simulink model "main"  (R2024a)
settings: Solver=VariableStepAuto  StartTime=0.0  StopTime=stop_time  RelTol=1e-3
values from neighbouring files (symbols this model uses):
  A_ca = sqrt(2)    [load_params.m]
  c = 299792458    [load_params.m]
  ca_code = 1    [load_params.m]
  code_repeat = 0.001    [load_params.m]
  data_repeat = 30    [load_params.m]
  df_Dop = 0    [load_params.m]
  dt_iono = 0    [load_params.m]
  dt_rec = 0.001    [load_params.m]
  dt_sv = 0    [load_params.m]
  dt_tropo = 0    [load_params.m]
  fB = 1.5e6    (= 1500000)    [load_params.m]
  fb = fB    (= 1500000)    [load_params.m]
  fc = 1.023e6    (= 1023000)    [load_params.m]
  fdata = 50    [load_params.m]
  ferr = 0    [load_params.m]
  fL1 = 1575.42e6    (= 1575420000)    [load_params.m]
  fs = 4e6    (= 4000000)    [load_params.m]
  nav_data = 1    [load_params.m]
  perr_rad = 0    [load_params.m]
  PIT = 0.010    (= 0.01)    [load_params.m]
  r_true_t0 = 20e6    (= 20000000)    [load_params.m]
  Ts = 1/fs    (= 2.5e-07)    [load_params.m]
undefined symbols (not defined in the file or in its folder): DiscIntNeverNeededParam
libraries: dspsrcs4 x2, commfilt2 x2
settings Model: Creator=Alireza  LastModifiedBy=Alireza

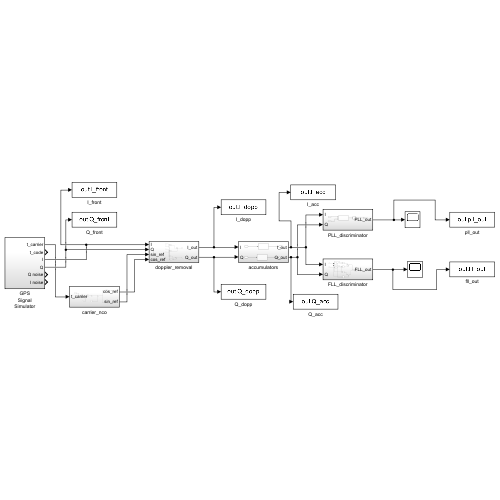
[thumbnail: Simulink's stored preview of the top-level diagram]
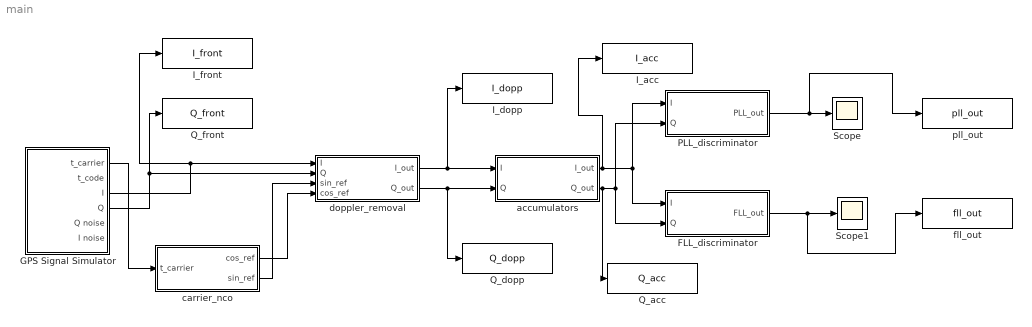
== system main ==
  FLL_discriminator : Subsystem
  GPS Signal Simulator : Subsystem
  I_acc : ToWorkspace  VariableName=I_acc  SampleTime=-1
  I_dopp : ToWorkspace  VariableName=I_dopp  SampleTime=-1
  I_front : ToWorkspace  VariableName=I_front  SampleTime=-1
  PLL_discriminator : Subsystem
  Q_acc : ToWorkspace  VariableName=Q_acc  SampleTime=-1
  Q_dopp : ToWorkspace  VariableName=Q_dopp  SampleTime=-1
  Q_front : ToWorkspace  VariableName=Q_front  SampleTime=-1
  Scope : Scope
  Scope1 : Scope
  accumulators : Subsystem
  carrier_nco : Subsystem
  doppler_removal : Subsystem
  fll_out : ToWorkspace  VariableName=fll_out  SampleTime=-1
  pll_out : ToWorkspace  VariableName=pll_out  SampleTime=-1
  wires:
  carrier_nco/1(cos_ref) -> doppler_removal/4(cos_ref)
  carrier_nco/2(sin_ref) -> doppler_removal/3(sin_ref)
  doppler_removal/1(I_out) -> I_dopp/1, accumulators/1(I)
  doppler_removal/2(Q_out) -> Q_dopp/1, accumulators/2(Q)
  accumulators/1(I_out) -> I_acc/1, FLL_discriminator/1(I), PLL_discriminator/1(I)
  accumulators/2(Q_out) -> Q_acc/1, FLL_discriminator/2(Q), PLL_discriminator/2(Q)
  GPS Signal Simulator/3(I) -> I_front/1, doppler_removal/1(I)
  GPS Signal Simulator/4(Q) -> Q_front/1, doppler_removal/2(Q)
  GPS Signal Simulator/1(t_carrier) -> carrier_nco/1(t_carrier)
  PLL_discriminator/1(PLL_out) -> pll_out/1, Scope/1
  FLL_discriminator/1(FLL_out) -> fll_out/1, Scope1/1

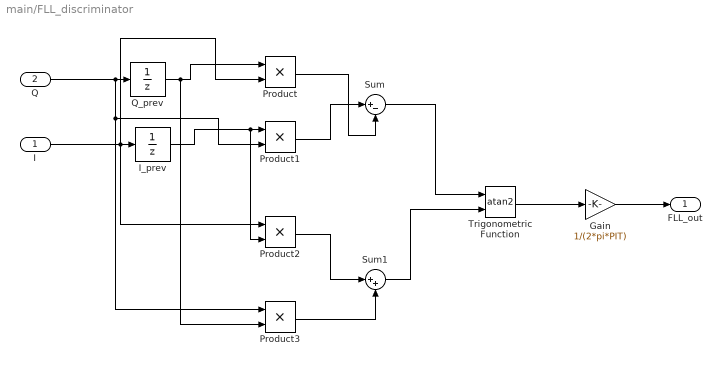
== system main/FLL_discriminator ==
  I : Inport
  Q : Inport  Port=2
  Gain : Gain  Gain=1/(2*pi*PIT)
  I_prev : UnitDelay  SampleTime=-1  HasFrameUpgradeWarning=on
  Product{,1..3} (4 alike) : Product
  Q_prev : UnitDelay  SampleTime=-1  HasFrameUpgradeWarning=on
  Sum : Sum  Inputs=|+-
  Sum1 : Sum  Inputs=|++
  Trigonometric Function : Trigonometry  Operator=atan2
  FLL_out : Outport
  wires:
  I/1 -> Product/2, I_prev/1, Product2/1
  Q/1 -> Product1/2, Product3/1, Q_prev/1
  I_prev/1 -> Product2/2, Product1/1
  Q_prev/1 -> Product3/2, Product/1
  Product1/1 -> Sum/1
  Product/1 -> Sum/2
  Product2/1 -> Sum1/1
  Product3/1 -> Sum1/2
  Sum/1 -> Trigonometric Function/1
  Sum1/1 -> Trigonometric Function/2
  Trigonometric Function/1 -> Gain/1
  Gain/1 -> FLL_out/1

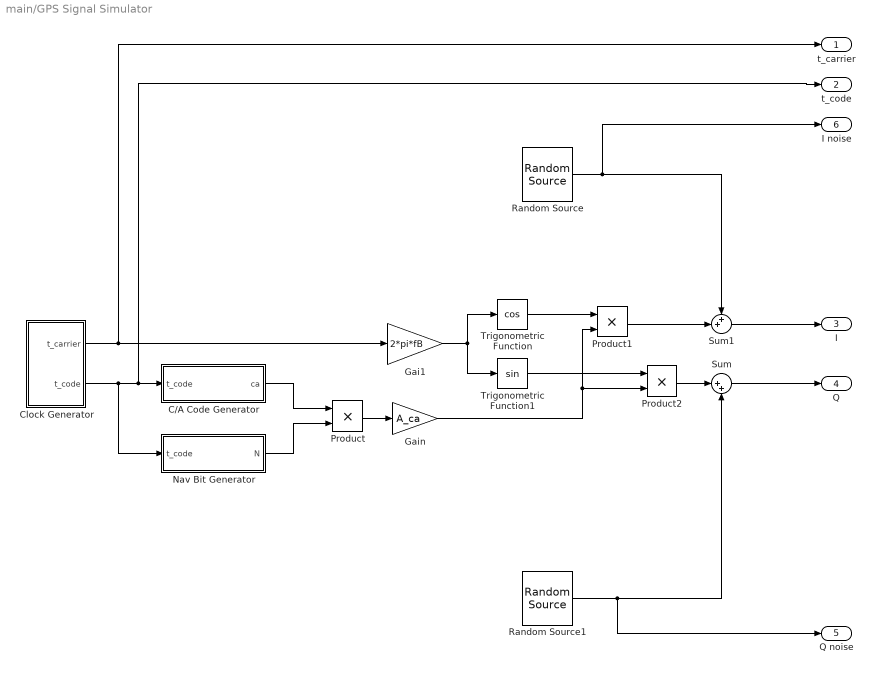
== system main/GPS Signal Simulator ==
  C/A Code Generator : Subsystem
  Clock Generator : Subsystem
  Gai1 : Gain  Gain=2*pi*fB
  Gain : Gain  Gain=A_ca
  Nav Bit Generator : Subsystem
  Product : Product  RndMeth=Zero
  Product1 : Product  RndMeth=Zero
  Product2 : Product  RndMeth=Zero
  Random Source : dspsrcs4/Random Source  SrcType=Gaussian  MinVal=0  MaxVal=1  MeanVal=0  VarVal=Pn  RepMode=Specify seed  rawSeed=1  IsInherit=off  SampTime=Ts  SampFrame=1  OutComplex=Real  DataType=double  SimulateUsing=Interpreted execution
  Random Source1 : dspsrcs4/Random Source  SrcType=Gaussian  MinVal=0  MaxVal=1  MeanVal=0  VarVal=Pn  RepMode=Specify seed  rawSeed=2  IsInherit=off  SampTime=Ts  SampFrame=1  OutComplex=Real  DataType=double  SimulateUsing=Interpreted execution
  Sum : Sum  Inputs=|++
  Sum1 : Sum  Inputs=++|
  Trigonometric Function : Trigonometry  Operator=cos
  Trigonometric Function1 : Trigonometry
  t_carrier : Outport
  t_code : Outport  Port=2
  I : Outport  Port=3
  Q : Outport  Port=4
  Q noise : Outport  Port=5
  I noise : Outport  Port=6
  wires:
  Clock Generator/2(t_code) -> Nav Bit Generator/1(t_code), C/A Code Generator/1(t_code), t_code/1
  C/A Code Generator/1(ca) -> Product/1
  Nav Bit Generator/1(N) -> Product/2
  Product/1 -> Gain/1
  Clock Generator/1(t_carrier) -> Gai1/1, t_carrier/1
  Gai1/1 -> Trigonometric Function1/1, Trigonometric Function/1
  Gain/1 -> Product1/2, Product2/2
  Trigonometric Function/1 -> Product1/1
  Trigonometric Function1/1 -> Product2/1
  Random Source1/1 -> Sum/2, Q noise/1
  Random Source/1 -> Sum1/1, I noise/1
  Sum/1 -> Q/1
  Sum1/1 -> I/1
  Product1/1 -> Sum1/2
  Product2/1 -> Sum/1

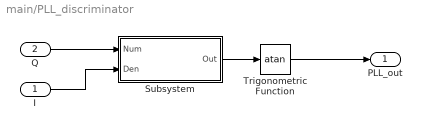
== system main/PLL_discriminator ==
  I : Inport
  Q : Inport  Port=2
  Subsystem : Subsystem
  Trigonometric Function : Trigonometry  Operator=atan
  PLL_out : Outport
  wires:
  Subsystem/1(Out) -> Trigonometric Function/1
  Trigonometric Function/1 -> PLL_out/1
  Q/1 -> Subsystem/1(Num)
  I/1 -> Subsystem/2(Den)

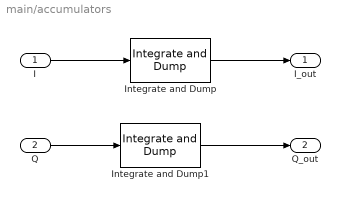
== system main/accumulators ==
  I : Inport
  Q : Inport  Port=2
  Integrate and Dump : commfilt2/Integrate and Dump  obssamples=PIT*fs  offsetsamples=0  nodump=off  roundingMode=Floor  overflowMode=off  outputDataTypeStr=Inherit: Same as accumulator  outputLastDataTypeStr=Inherit: Same as accumulator
  Integrate and Dump1 : commfilt2/Integrate and Dump  obssamples=PIT*fs  offsetsamples=0  nodump=off  roundingMode=Floor  overflowMode=off  outputDataTypeStr=Inherit: Same as accumulator  outputLastDataTypeStr=Inherit: Same as accumulator
  I_out : Outport
  Q_out : Outport  Port=2
  wires:
  I/1 -> Integrate and Dump/1
  Integrate and Dump/1 -> I_out/1
  Integrate and Dump1/1 -> Q_out/1
  Q/1 -> Integrate and Dump1/1

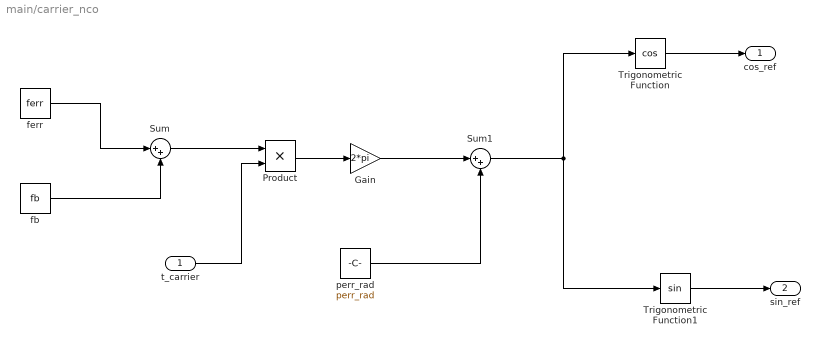
== system main/carrier_nco ==
  t_carrier : Inport
  Gain : Gain  Gain=2*pi
  Product : Product
  Sum : Sum  Inputs=|++
  Sum1 : Sum  Inputs=|++
  Trigonometric Function : Trigonometry  Operator=cos
  Trigonometric Function1 : Trigonometry
  fb : Constant  Value=fb
  ferr : Constant  Value=ferr
  perr_rad : Constant  Value=perr_rad
  cos_ref : Outport
  sin_ref : Outport  Port=2
  wires:
  Trigonometric Function1/1 -> sin_ref/1
  t_carrier/1 -> Product/2
  Sum1/1 -> Trigonometric Function1/1, Trigonometric Function/1
  Trigonometric Function/1 -> cos_ref/1
  perr_rad/1 -> Sum1/2
  Gain/1 -> Sum1/1
  fb/1 -> Sum/2
  Product/1 -> Gain/1
  ferr/1 -> Sum/1
  Sum/1 -> Product/1

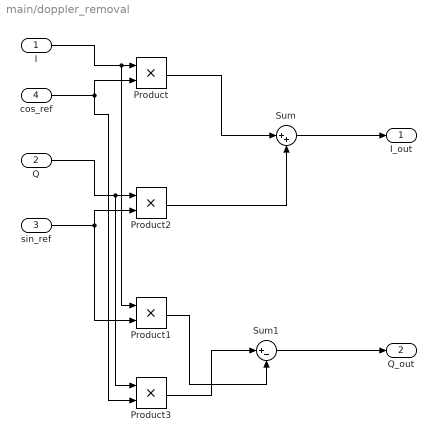
== system main/doppler_removal ==
  I : Inport
  Q : Inport  Port=2
  sin_ref : Inport  Port=3
  cos_ref : Inport  Port=4
  Product{,1..3} (4 alike) : Product
  Sum : Sum  Inputs=|++
  Sum1 : Sum  Inputs=|+-
  I_out : Outport
  Q_out : Outport  Port=2
  wires:
  I/1 -> Product1/1, Product/1
  cos_ref/1 -> Product3/2, Product/2
  Q/1 -> Product2/1, Product3/1
  sin_ref/1 -> Product1/2, Product2/2
  Product/1 -> Sum/1
  Product2/1 -> Sum/2
  Sum/1 -> I_out/1
  Sum1/1 -> Q_out/1
  Product3/1 -> Sum1/1
  Product1/1 -> Sum1/2

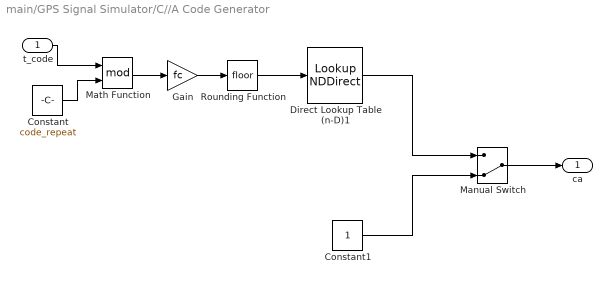
== system main/GPS Signal Simulator/C//A Code Generator ==
  t_code : Inport
  Constant : Constant  Value=code_repeat
  Constant1 : Constant
  Direct Lookup Table (n-D)1 : LookupNDDirect  NumberOfTableDimensions=1  Table=ca_code
  Gain : Gain  Gain=fc
  Manual Switch : ManualSwitch  CurrentSetting=0
  Math Function : Math  Operator=mod  SignedPower=on
  Rounding Function : Rounding
  ca : Outport
  wires:
  Constant/1 -> Math Function/2
  Math Function/1 -> Gain/1
  Gain/1 -> Rounding Function/1
  Rounding Function/1 -> Direct Lookup Table (n-D)1/1
  t_code/1 -> Math Function/1
  Direct Lookup Table (n-D)1/1 -> Manual Switch/1
  Constant1/1 -> Manual Switch/2
  Manual Switch/1 -> ca/1

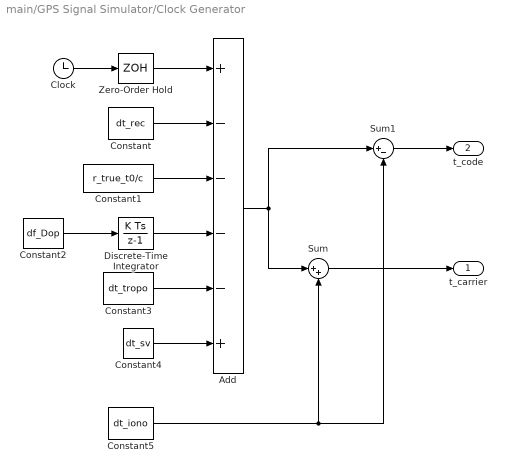
== system main/GPS Signal Simulator/Clock Generator ==
  Add : Sum  Inputs=+----+
  Clock : Clock
  Constant : Constant  Value=dt_rec
  Constant1 : Constant  Value=r_true_t0/c
  Constant2 : Constant  Value=df_Dop
  Constant3 : Constant  Value=dt_tropo
  Constant4 : Constant  Value=dt_sv
  Constant5 : Constant  Value=dt_iono
  Discrete-Time Integrator : DiscreteIntegrator  gainval=1/fL1  SampleTime=Ts  ICPrevOutput=DiscIntNeverNeededParam  ICPrevScaledInput=DiscIntNeverNeededParam
  Sum : Sum  Inputs=|++
  Sum1 : Sum  Inputs=|+-
  Zero-Order Hold : ZeroOrderHold  SampleTime=Ts
  t_carrier : Outport
  t_code : Outport  Port=2
  wires:
  Clock/1 -> Zero-Order Hold/1
  Constant/1 -> Add/2
  Constant1/1 -> Add/3
  Constant2/1 -> Discrete-Time Integrator/1
  Discrete-Time Integrator/1 -> Add/4
  Constant3/1 -> Add/5
  Zero-Order Hold/1 -> Add/1
  Constant4/1 -> Add/6
  Add/1 -> Sum/1, Sum1/1
  Constant5/1 -> Sum/2, Sum1/2
  Sum1/1 -> t_code/1
  Sum/1 -> t_carrier/1

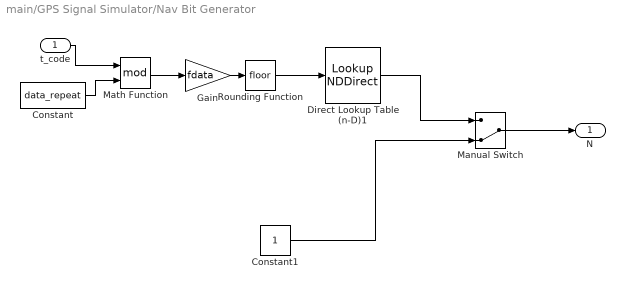
== system main/GPS Signal Simulator/Nav Bit Generator ==
  t_code : Inport
  Constant : Constant  Value=data_repeat
  Constant1 : Constant
  Direct Lookup Table (n-D)1 : LookupNDDirect  NumberOfTableDimensions=1  Table=nav_data
  Gain : Gain  Gain=fdata
  Manual Switch : ManualSwitch  CurrentSetting=0
  Math Function : Math  Operator=mod  SignedPower=on
  Rounding Function : Rounding
  N : Outport
  wires:
  Constant/1 -> Math Function/2
  Math Function/1 -> Gain/1
  Gain/1 -> Rounding Function/1
  Rounding Function/1 -> Direct Lookup Table (n-D)1/1
  t_code/1 -> Math Function/1
  Direct Lookup Table (n-D)1/1 -> Manual Switch/1
  Constant1/1 -> Manual Switch/2
  Manual Switch/1 -> N/1

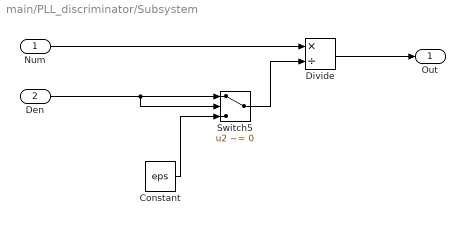
== system main/PLL_discriminator/Subsystem ==
  Num : Inport
  Den : Inport  Port=2
  Constant : Constant  Value=eps  SampleTime=-1
  Divide : Product  Inputs=*/
  Switch5 : Switch  Criteria=u2 ~= 0  ZeroCross=off  SaturateOnIntegerOverflow=off  InputSameDT=off
  Out : Outport
  wires:
  Num/1 -> Divide/1
  Constant/1 -> Switch5/3
  Switch5/1 -> Divide/2
  Den/1 -> Switch5/1, Switch5/2
  Divide/1 -> Out/1
